simulink library "dis"  (Simulink 8.1)
settings: Solver=ode45  StartTime=0.0  StopTime=10.0  RelTol=1e-3
settings Model: Creator=xsellart  LastModifiedBy=AT015555

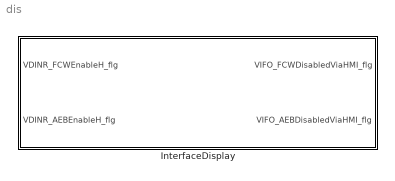
== system dis ==
  InterfaceDisplay : Subsystem

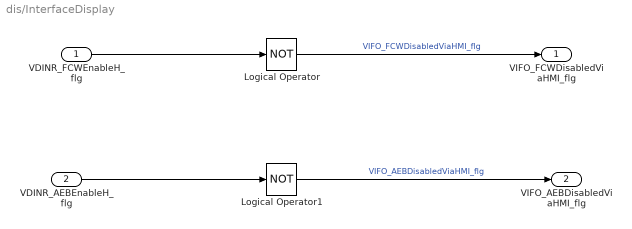
== system dis/InterfaceDisplay ==
  VDINR_FCWEnableH_flg : Inport
  VDINR_AEBEnableH_flg : Inport  Port=2
  Logical Operator : Logic  Operator=NOT  AllPortsSameDT=off  OutDataTypeStr=boolean
  Logical Operator1 : Logic  Operator=NOT  AllPortsSameDT=off  OutDataTypeStr=boolean
  VIFO_FCWDisabledViaHMI_flg : Outport
  VIFO_AEBDisabledViaHMI_flg : Outport  Port=2
  wires:
  VDINR_AEBEnableH_flg/1 -> Logical Operator1/1
  Logical Operator1/1 -> VIFO_AEBDisabledViaHMI_flg/1  "VIFO_AEBDisabledViaHMI_flg"
  Logical Operator/1 -> VIFO_FCWDisabledViaHMI_flg/1  "VIFO_FCWDisabledViaHMI_flg"
  VDINR_FCWEnableH_flg/1 -> Logical Operator/1
